simulink model "GalvoModel_v42"  (R2013a)
settings: Solver=ode45  StartTime=0.0  StopTime=10.0  MaxStep=1e-4  RelTol=1e-3
InitFcn:
  | param=evalin('base','param;');
  | 
  | JR=str2num(param.JR);
  | KMT=str2num(param.KMT);
  | Rc=str2num(param.Rc);
  | Lc=str2num(param.Lc);
  | KFR=str2num(param.KFR);
  | KTB=str2num(param.KTB);
  | KBM=str2num(param.KBM);
  | Rsh=str2num(param.Rsh);
StartFcn:
  | sprintf('Info (%s):\nKTB = %.1e\nKBM = %.1e\n', gcs, KTB, KBM)
model workspace (MATLAB code in the model file):
  | %param=evalin('base','loadGalvoParam(4);');
  | param=evalin('base','param;');
  | 
  | JR=str2num(param.JR);
  | KMT=str2num(param.KMT);
  | Rc=str2num(param.Rc);
  | Lc=str2num(param.Lc);
  | KFR=str2num(param.KFR);
  | KTB=str2num(param.KTB);
  | KBM=str2num(param.KBM);
  | Rsh=str2num(param.Rsh);
settings Model: Creator=mainster  LastModifiedBy=mainster
settings OptimizationCC: InlineParams=on

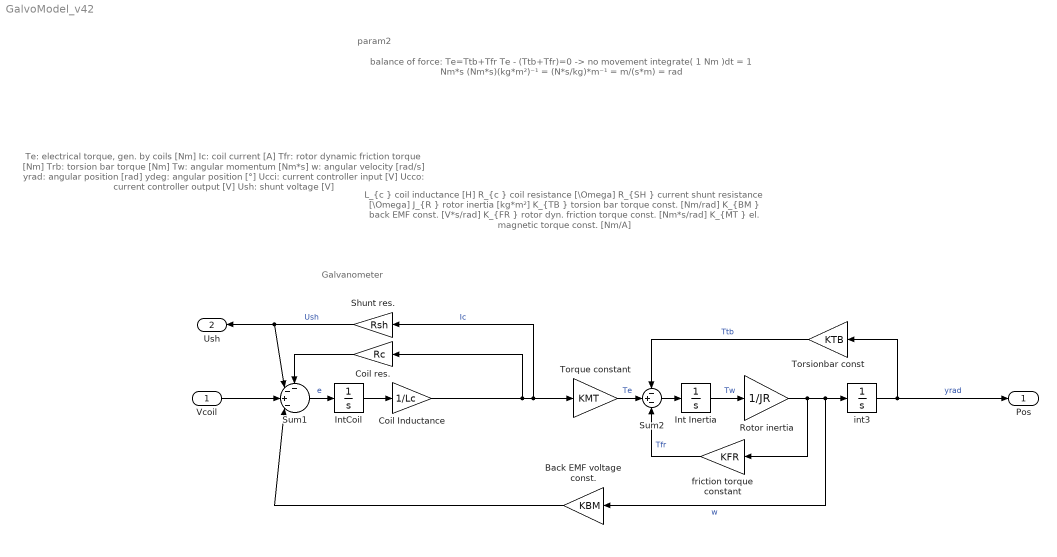
== system GalvoModel_v42 ==
  note: param2
  note: Galvanometer
  note: Te: 		electrical torque, gen. by coils		[Nm]
      |  Ic: 			coil current							[A]
      |  Tfr:		rotor dynamic friction torque 		[Nm]
      |  Trb:		torsion bar torque					[Nm]
      |  Tw:		angular momentum				[Nm*s]
      |  w:			angular velocity 					[rad/s]
      |  yrad:		angular position 					[rad]
      |  ydeg:		angular position 					[°]
      |  Ucci:		current controller input				[V]
      |  Ucco:		current controller output			[V]
      |  Ush:		shunt voltage						[V]
  note: L_{c  }	coil inductance 							[H]
      |  R_{c  }	coil resistance							[\Omega]
      |  R_{SH }	current shunt resistance				[\Omega]
      |  J_{R  }	rotor inertia 							[kg*m²]
      |  K_{TB }	torsion bar torque const. 			[Nm/rad]
      |  K_{BM }	back EMF const.							[V*s/rad]
      |  K_{FR }	rotor dyn. friction torque const.	[Nm*s/rad]
      |  K_{MT }	el. magnetic torque const.			[Nm/A]
  note: balance of force: 	Te=Ttb+Tfr
      | 					Te - (Ttb+Tfr)=0  ->  no movement
      |
      |  integrate( 1 Nm )dt = 1 Nm*s
      |  (Nm*s)(kg*m²)⁻¹ = (N*s/kg)*m⁻¹ = m/(s*m) = rad
  Vcoil : Inport
  Back EMF voltage const. : Gain  Gain=KBM
  Coil Inductance : Gain  Gain=1/Lc
  Coil res. : Gain  Gain=Rc
  Int Inertia : Integrator
  IntCoil : Integrator
  Rotor inertia : Gain  Gain=1/JR
  Shunt res. : Gain  Gain=Rsh
  Sum1 : Sum  Inputs=--+-|
  Sum2 : Sum  Inputs=-+-
  Torque constant : Gain  Gain=KMT
  Torsionbar const : Gain  Gain=KTB
  friction torque constant : Gain  Gain=KFR
  int3 : Integrator
  Pos : Outport
  Ush : Outport  Port=2
  wires:
  Shunt res./1 -> Ush/1, Sum1/2  "Ush"
  Coil res./1 -> Sum1/1
  Vcoil/1 -> Sum1/3
  Back EMF voltage const./1 -> Sum1/4
  int3/1 -> Pos/1, Torsionbar const/1  "yrad"
  Torque constant/1 -> Sum2/2  "Te"
  Coil Inductance/1 -> Shunt res./1, Torque constant/1, Coil res./1  "Ic"
  Torsionbar const/1 -> Sum2/1  "Ttb"
  IntCoil/1 -> Coil Inductance/1
  Sum1/1 -> IntCoil/1  "e"
  Int Inertia/1 -> Rotor inertia/1  "Tw"
  Sum2/1 -> Int Inertia/1
  Rotor inertia/1 -> int3/1, Back EMF voltage const./1, friction torque constant/1  "w"
  friction torque constant/1 -> Sum2/3  "Tfr"
